simulink model "ModeAdjust"  (R2018b)
settings: Solver=FixedStepDiscrete  StartTime=0.0  StopTime=inf  FixedStep=0.01  RelTol=1e-3
undefined symbols (not defined in the file or in its folder): IfKeSMSbSeatMovBkRclnEnable_Val, IfKeSMSbSeatMovFrwdBkwdEnable_Val, IfKeSMSbSeatMovFtrstEnable_Val, IfKeSMSbSeatMovHdrstFrwdBkwdEnable_Val, IfKeSMSbSeatMovHdUpwdDnwdEnable_Val, IfKeSMSbSeatMovLgrstEnable_Val, IfKeSMSbSeatMovLtwdRtwdEnable_Val, IfVeSMSeStNumConfig, KeSMSbArmscreenMovEnable_Val, KeSMSbSeatMovLgrstExpdEnable_Val, KeSMSuFirstRwStBackPosDelta_Val, KeSMSuFirstRwStBackPosTolr_Val, KeSMSuFirstRwStCushFrntPosDelta_Val, KeSMSuFirstRwStCushFrntPosTolr_Val, KeSMSuFirstRwStCushRePosDelta_Val, KeSMSuFirstRwStCushRePosTolr_Val, KeSMSuFirstRwStFootrestPosDelta_Val, KeSMSuFirstRwStFootrestPosTolr_Val, KeSMSuFirstRwStFwdBkwdPosDelta_Val, KeSMSuFirstRwStFwdBkwdPosTolr_Val, KeSMSuMdMotFinshdTm_Val, KeSMSuMdRetryTm1_Val, KeSMSuModeReqDurgTm_Val, KeSMSuSecRwStArmTochPosDelta_Val, KeSMSuSecRwStArmTochPosTolr_Val, KeSMSuSecRwStBackPosDelta_Val, KeSMSuSecRwStBackPosTolr_Val, KeSMSuSecRwStFtrstUpwdDnwdPosDelta_Val, KeSMSuSecRwStFtrstUpwdDnwdPosTolr_Val, KeSMSuSecRwStFwdBkwdPosDelta_Val, KeSMSuSecRwStFwdBkwdPosTolr_Val, KeSMSuSecRwStHeadrestFwdBkwdPosDelta_Val, KeSMSuSecRwStHeadrestFwdBkwdPosTolr_Val, KeSMSuSecRwStHeadrestUpwdDwnwdPosDelta_Val, KeSMSuSecRwStHeadrestUpwdDwnwdPosTolr_Val, KeSMSuSecRwStLegrestInOutPosDelta_Val, KeSMSuSecRwStLegrestInOutPosTolr_Val, KeSMSuSecRwStLegrestUpwdDwnwdPosDelta_Val, KeSMSuSecRwStLegrestUpwdDwnwdPosTolr_Val, KeSMSuSecRwStLwdRwdPosDelta_Val, KeSMSuSecRwStLwdRwdPosTolr_Val, KeSMSuSecRwStVIPFtrstRefAngle_Val, KeSMSuThirdRwStFwdBkwdPosDelta_Val, KeSMSuThirdRwStFwdBkwdPosTolr_Val, KeSMSuThrdRwCushFoldPosDelta_Val, KeSMSuThrdRwCushFoldPosTolr_Val, KeSMSuThrdRwStBackPosDelta_Val, KeSMSuThrdRwStBackPosTolr_Val, KeSMSw4SLegrstCloseMdSecRwLtStFtrstUpwdDnwdPos_Val, KeSMSw4SLegrstCloseMdSecRwLtStFtrstUpwdDnwdPosMax_Val, KeSMSw4SLegrstCloseMdSecRwLtStFtrstUpwdDnwdPosMin_Val, KeSMSw4SLegrstCloseMdSecRwLtStLgrstOtwdInwdPos_Val, KeSMSw4SLegrstCloseMdSecRwLtStLgrstOtwdInwdPosMax_Val, KeSMSw4SLegrstCloseMdSecRwLtStLgrstOtwdInwdPosMin_Val, KeSMSw4SLegrstCloseMdSecRwLtStLgrstUpwdDnwdPos_Val, KeSMSw4SLegrstCloseMdSecRwLtStLgrstUpwdDnwdPosMax_Val, KeSMSw4SLegrstCloseMdSecRwLtStLgrstUpwdDnwdPosMin_Val, KeSMSw4SLegrstCloseMdSecRwRtStFtrstUpwdDnwdPos_Val, KeSMSw4SLegrstCloseMdSecRwRtStFtrstUpwdDnwdPosMax_Val, KeSMSw4SLegrstCloseMdSecRwRtStFtrstUpwdDnwdPosMin_Val ... (+1138)
libraries: Lib x401
(part 12 of 35)

== system ModeAdjust/ModeAdjustRunnable_sys/ModeAdjust/AcsMdEntry/R2Rt ==
  note: /*短期措施：二右扶手屏配置信号原先的短期措施blost inout被头枕前后占用，暂时默认扶手屏始终配置，等46数据库再连线*/
  note: %1锁，2未锁
  Mode_Trig : Inport
  Step1En : Inport  Port=2
  Step2En : Inport  Port=3
  SecRwRtStPoss : Inport  Port=4
  SecRwRtStPossV : Inport  Port=5
  SecRwRtStChldLkRsp_L : Inport  Port=6
  ModeStCalib_2R : Inport  Port=7
  StConfig : Inport  Port=8
  isR2RtSeatOccupied : Inport  Port=9
  AND : Logic  AllPortsSameDT=off  OutDataTypeStr=boolean
  Bus Creator : BusCreator  Inputs=9  OutDataTypeStr=Bus: SecRwRtSeatPos
  Bus Selector : BusSelector  OutputSignals=IfVeSMSuSecRwRtStBkReclnUpwdDnwdPos_Val_read,IfVeSMSuSecRwRtStFrwdBkwdPos_Val_read,IfVeSMSuSecRwRtStHPassStUpwdDnwdPos_Val_read,IfVeSMSuSecRwRtStLgrstUpwdDnwdPos_Val_read,IfVeSMSuSecRwRtStLtwdRtwdPos_Val_read,SecRwRtStArmScrnPos_Val_read
  Bus Selector1 : BusSelector  OutputSignals=IfVeSMSuSecRwRtStBkReclnUpwdDnwdPosV_Val_read,IfVeSMSuSecRwRtStFrwdBkwdPosV_Val_read,IfVeSMSuSecRwRtStHPassStUpwdDnwdPosV_Val_read,IfVeSMSuSecRwRtStLgrstUpwdDnwdPosV_Val_read,IfVeSMSuSecRwRtStLtwdRtwdPosV_Val_read,SecRwRtStArmScrnPosV_Val_read
  Bus Selector2 : BusSelector  OutputSignals=ArmScrnPos,ArmScrnPosMax,ArmScrnPosMin,BkReclnUpwdDnwdPos,BkReclnUpwdDnwdPosMax,BkReclnUpwdDnwdPosMin,FrwdBkwdPos,FrwdBkwdPosMax,FrwdBkwdPosMin,HdrstUpwdPos,HdrstUpwdPosMax,HdrstUpwdPosMin,LgrstUpwdPos,LgrstUpwdPosMax,LgrstUpwdPosMin,LtwdRtwdPos,LtwdRtwdPosMax,LtwdRtwdPosMin
  Bus Selector3 : BusSelector  OutputSignals=AcsEntrySecRwRtSt
  Bus Selector4 : BusSelector  OutputSignals=BkReclnUpwdDnwdMovConfig,ArmTouchMovConfig,FrwdBkwdMovConfig,LgrstUpwdMovConfig,LtwdRtwdMovConfig
  Logical Operator1 : Logic  Inputs=3  AllPortsSameDT=off  OutDataTypeStr=boolean
  Logical Operator2 : Logic  Inputs=3  AllPortsSameDT=off  OutDataTypeStr=boolean
  Logical Operator3 : Logic  AllPortsSameDT=off  OutDataTypeStr=boolean
  Logical Operator4 : Logic  AllPortsSameDT=off  OutDataTypeStr=boolean
  Logical Operator5 : Logic  Operator=OR  AllPortsSameDT=off  OutDataTypeStr=boolean
  Logical Operator6 : Logic  AllPortsSameDT=off  OutDataTypeStr=boolean
  NOT : Logic  Operator=NOT  AllPortsSameDT=off  OutDataTypeStr=boolean
  PA_KeSMSuMdMotFinshdTm_Val : Constant  Value=KeSMSuMdMotFinshdTm_Val
  PA_KeSMSuMdRetryTm1_Val : Constant  Value=KeSMSuMdRetryTm1_Val
  PA_KeSMSuModeReqDurgTm_Val : Constant  Value=KeSMSuModeReqDurgTm_Val
  PA_KeSMSuSecRwStArmTochPosDelta_Val : Constant  Value=KeSMSuSecRwStArmTochPosDelta_Val
  PA_KeSMSuSecRwStBackPosDelta_Val : Constant  Value=KeSMSuSecRwStBackPosDelta_Val
  PA_KeSMSuSecRwStFwdBkwdPosDelta_Val : Constant  Value=KeSMSuSecRwStFwdBkwdPosDelta_Val
  PA_KeSMSuSecRwStLegrestUpwdDwnwdPosDelta_Val : Constant  Value=KeSMSuSecRwStLegrestUpwdDwnwdPosDelta_Val
  PA_KeSMSuSecRwStLwdRwdPosDelta_Val : Constant  Value=KeSMSuSecRwStLwdRwdPosDelta_Val
  PA_KeSMSwDltTrgtPos_Val{1,4..5,7..9,11,14,16} (9 alike) : Constant  Value=0  OutDataTypeStr=boolean
  PA_KeSMSwDltTrgtPos_Val{3,6,10,12,15,17,19..22} (10 alike) : Constant  Value=KeSMSwPosInvalidVal_Val
  PA_KeSMSwDltTrgtPos_Val18 : Constant  Value=3  OutDataTypeStr=uint8
  PA_KeSMSwDltTrgtPos_Val2 : Constant  Value=SeatChldLkSt.ChldLkSt_Unlock
  PA_KeSMSwDltTrgtPos_Val23 : Constant  Value=2  OutDataTypeStr=uint8
  PA_KeSMSwSecRwRtStEasyEntryCllsnPt_Val : Constant  Value=KeSMSwSecRwRtStEasyEntryCllsnPt_Val
  R2RtSt_BkReclnUpwdDnwd_Step1 : Lib/CommonUsed  SystemSampleTime=-1
  R2RtSt_FrwdBkwd_Step2 : Lib/CommonUsed  SystemSampleTime=-1
  R2RtSt_LgrstUpwd_Step1 : Lib/CommonUsed  SystemSampleTime=-1
  R2Rt_LtwdRtwd_Step2 : Lib/CommonUsed  SystemSampleTime=-1
  Relational Operator : RelationalOperator  Operator=~=  OutDataTypeStr=boolean  RndMeth=Simplest
  Relational Operator1 : RelationalOperator  Operator=<=  OutDataTypeStr=boolean  RndMeth=Simplest
  Relational Operator2 : RelationalOperator  Operator=~=  OutDataTypeStr=boolean  RndMeth=Simplest
  SecRwRtStArmScrnPos_Step1 : Lib/CommonUsed  SystemSampleTime=-1
  Switch : Switch  Criteria=u2 ~= 0
  R2RtSt_Step1_ini : Outport
  R2RtSt_Step2_ini : Outport  Port=2
  R2Rt_Step1_done : Outport  Port=3
  R2Rt_Step2_done : Outport  Port=4
  R2Rt_TrgtPoss : Outport  Port=5  VectorParamsAs1DForOutWhenUnconnected=on
  R2Rt_SpdCtrl : Outport  Port=6
  wires:
  R2RtSt_LgrstUpwd_Step1/4 -> [Step1done_2]
  R2RtSt_LgrstUpwd_Step1/3 -> [R2RtSt_LgrstUpwd_TarPos]
  R2RtSt_LgrstUpwd_Step1/2 -> [Step1_2_ArrivedTarPos]
  [Tick] -> R2RtSt_LgrstUpwd_Step1/11
  PA_KeSMSwDltTrgtPos_Val12/1 -> R2RtSt_LgrstUpwd_Step1/10
  PA_KeSMSwDltTrgtPos_Val11/1 -> R2RtSt_LgrstUpwd_Step1/9
  [SecRwRtStLgrstUpwdDnwdPosV] -> R2RtSt_LgrstUpwd_Step1/8
  [KeSMSuSecRwStLegrestUpwdDwnwdPosDelta_Val] -> R2RtSt_LgrstUpwd_Step1/7
  [SecRwRtStBkReclnUpwdDnwdPosV] -> R2RtSt_BkReclnUpwdDnwd_Step1/8
  [SecRwRtStLgrstUpwdDnwdPos] -> R2RtSt_LgrstUpwd_Step1/3
  [K_LgrstUpwdPos] -> R2RtSt_LgrstUpwd_Step1/6
  [K_LgrstUpwdPosMax] -> R2RtSt_LgrstUpwd_Step1/5
  [K_LgrstUpwdPosMin] -> R2RtSt_LgrstUpwd_Step1/4
  [Step1En] -> R2RtSt_LgrstUpwd_Step1/2
  [Trig] -> R2RtSt_LgrstUpwd_Step1/1
  Relational Operator/1 -> [ChildLocker]
  PA_KeSMSwDltTrgtPos_Val2/1 -> Relational Operator/2
  SecRwRtStChldLkRsp_L/1 -> Relational Operator/1
  R2RtSt_FrwdBkwd_Step2/4 -> [Step2done_1]
  [Tick] -> R2RtSt_FrwdBkwd_Step2/11
  [Tick] -> R2RtSt_BkReclnUpwdDnwd_Step1/11
  PA_KeSMSwDltTrgtPos_Val6/1 -> R2RtSt_FrwdBkwd_Step2/10
  PA_KeSMSwDltTrgtPos_Val14/1 -> R2RtSt_FrwdBkwd_Step2/9
  [ChildLocker] -> R2RtSt_BkReclnUpwdDnwd_Step1/9
  [SecRwRtStFrwdBkwdPosV] -> R2RtSt_FrwdBkwd_Step2/8
  [K_FrwdBkwdPos] -> R2RtSt_FrwdBkwd_Step2/6
  [Step2En] -> R2RtSt_FrwdBkwd_Step2/2
  [Trig] -> R2RtSt_FrwdBkwd_Step2/1
  [Step1En] -> R2RtSt_BkReclnUpwdDnwd_Step1/2
  R2RtSt_BkReclnUpwdDnwd_Step1/4 -> [Step1done_1]
  R2RtSt_BkReclnUpwdDnwd_Step1/3 -> [R2RtSt_BkReclnUpwdDnwd_TarPos]
  PA_KeSMSwDltTrgtPos_Val3/1 -> R2RtSt_BkReclnUpwdDnwd_Step1/10
  [K_BkReclnUpwdDnwdPos] -> R2RtSt_BkReclnUpwdDnwd_Step1/6
  [SecRwRtStBkReclnUpwdDnwdPos] -> R2RtSt_BkReclnUpwdDnwd_Step1/3
  R2RtSt_BkReclnUpwdDnwd_Step1/2 -> [Step1_1_ArrivedTarPos]
  [K_BkReclnUpwdDnwdPosMin] -> R2RtSt_BkReclnUpwdDnwd_Step1/4
  R2RtSt_FrwdBkwd_Step2/2 -> [Step2_1_ArrivedTarPos]
  R2RtSt_FrwdBkwd_Step2/1 -> [FrwdBkwd_inidone_Step2]
  [K_FrwdBkwdPosMin] -> R2RtSt_FrwdBkwd_Step2/4
  [KeSMSuSecRwStFwdBkwdPosDelta_Val] -> R2RtSt_FrwdBkwd_Step2/7
  [K_FrwdBkwdPosMax] -> R2RtSt_FrwdBkwd_Step2/5
  [SecRwRtStFrwdBkwdPos] -> R2RtSt_FrwdBkwd_Step2/3
  [KeSMSuSecRwStBackPosDelta_Val] -> R2RtSt_BkReclnUpwdDnwd_Step1/7
  Mode_Trig/1 -> [Trig]
  [Trig] -> R2RtSt_BkReclnUpwdDnwd_Step1/1
  [K_BkReclnUpwdDnwdPosMax] -> R2RtSt_BkReclnUpwdDnwd_Step1/5
  Bus Selector1/2 -> [SecRwRtStFrwdBkwdPosV]  "<IfVeSMSuSecRwRtStFrwdBkwdPosV_Val_read>"
  SecRwRtStPossV/1 -> Bus Selector1/1
  Bus Selector1/3 -> [SecRwRtStHPassStUpwdDnwdPosV]  "<IfVeSMSuSecRwRtStHPassStUpwdDnwdPosV_Val_read>"
  Bus Selector/4 -> [SecRwRtStLgrstUpwdDnwdPos]  "<IfVeSMSuSecRwRtStLgrstUpwdDnwdPos_Val_read>"
  Bus Selector1/1 -> [SecRwRtStBkReclnUpwdDnwdPosV]  "<IfVeSMSuSecRwRtStBkReclnUpwdDnwdPosV_Val_read>"
  Bus Selector/1 -> [SecRwRtStBkReclnUpwdDnwdPos]  "<IfVeSMSuSecRwRtStBkReclnUpwdDnwdPos_Val_read>"
  Bus Selector1/4 -> [SecRwRtStLgrstUpwdDnwdPosV]  "<IfVeSMSuSecRwRtStLgrstUpwdDnwdPosV_Val_read>"
  Bus Selector/5 -> [SecRwRtStLtwdRtwdPos]  "<IfVeSMSuSecRwRtStLtwdRtwdPos_Val_read>"
  SecRwRtStPoss/1 -> Bus Selector/1
  Bus Selector1/5 -> [SecRwRtStLtwdRtwdPosV]  "<IfVeSMSuSecRwRtStLtwdRtwdPosV_Val_read>"
  Bus Selector/3 -> [SecRwRtStHPassStUpwdDnwdPos]  "<IfVeSMSuSecRwRtStHPassStUpwdDnwdPos_Val_read>"
  Bus Selector/2 -> [SecRwRtStFrwdBkwdPos]  "<IfVeSMSuSecRwRtStFrwdBkwdPos_Val_read>"
  [SecRwRtStArmScrnPos] -> SecRwRtStArmScrnPos_Step1/3
  [SecRwRtStArmScrnPosV] -> SecRwRtStArmScrnPos_Step1/8
  [Trig] -> SecRwRtStArmScrnPos_Step1/1
  [Step1En] -> SecRwRtStArmScrnPos_Step1/2
  [K_ArmScrnPosMin] -> SecRwRtStArmScrnPos_Step1/4
  [K_ArmScrnPosMax] -> SecRwRtStArmScrnPos_Step1/5
  [K_ArmScrnPos] -> SecRwRtStArmScrnPos_Step1/6
  PA_KeSMSwDltTrgtPos_Val7/1 -> SecRwRtStArmScrnPos_Step1/9
  PA_KeSMSwDltTrgtPos_Val10/1 -> SecRwRtStArmScrnPos_Step1/10
  [Tick] -> SecRwRtStArmScrnPos_Step1/11
  R2RtSt_FrwdBkwd_Step2/3 -> [R2Rt_StFrwdBkwd_TarPos]
  [Step1done_1] -> Logical Operator2/1
  [Step1done_2] -> Logical Operator2/2
  [Step1done_3] -> Logical Operator2/3
  [SecRwRtStFrwdBkwdPos] -> Relational Operator1/1
  [Trig] -> R2Rt_LtwdRtwd_Step2/1
  [Step2done_1] -> Logical Operator5/1
  Logical Operator5/1 -> Logical Operator4/1
  Logical Operator4/1 -> R2Rt_LtwdRtwd_Step2/2
  Relational Operator1/1 -> Logical Operator5/2
  [Step2En] -> Logical Operator4/2
  [KeSMSuSecRwStArmTochPosDelta_Val] -> SecRwRtStArmScrnPos_Step1/7
  [SecRwRtStLtwdRtwdPos] -> R2Rt_LtwdRtwd_Step2/3
  [SecRwRtStLtwdRtwdPosV] -> R2Rt_LtwdRtwd_Step2/8
  [K_LtwdRtwdPosMin] -> R2Rt_LtwdRtwd_Step2/4
  [K_LtwdRtwdPosMax] -> R2Rt_LtwdRtwd_Step2/5
  [K_LtwdRtwdPos] -> R2Rt_LtwdRtwd_Step2/6
  [KeSMSuSecRwStLwdRwdPosDelta_Val] -> R2Rt_LtwdRtwd_Step2/7
  PA_KeSMSwDltTrgtPos_Val16/1 -> R2Rt_LtwdRtwd_Step2/9
  PA_KeSMSwDltTrgtPos_Val17/1 -> R2Rt_LtwdRtwd_Step2/10
  [Tick] -> R2Rt_LtwdRtwd_Step2/11
  R2Rt_LtwdRtwd_Step2/3 -> [R2Rt_LtwdRtwd_TarPos]
  R2Rt_LtwdRtwd_Step2/1 -> [LtwdRtwd_inidone_Step2]
  R2Rt_LtwdRtwd_Step2/2 -> [Step2_2_ArrivedTarPos]
  R2Rt_LtwdRtwd_Step2/4 -> [Step2done_2]
  R2RtSt_BkReclnUpwdDnwd_Step1/1 -> [ReclnUpwdDnwd_Step1_ini]
  R2RtSt_LgrstUpwd_Step1/1 -> [LgrstUpwd_Step1_ini]
  [ReclnUpwdDnwd_Step1_ini] -> Logical Operator1/1
  [LgrstUpwd_Step1_ini] -> Logical Operator1/2
  [LtStArmScrn_Step1_ini] -> Logical Operator1/3
  Logical Operator1/1 -> R2RtSt_Step1_ini/1
  [FrwdBkwd_inidone_Step2] -> Logical Operator6/1
  [LtwdRtwd_inidone_Step2] -> Logical Operator6/2
  Logical Operator6/1 -> R2RtSt_Step2_ini/1
  Logical Operator2/1 -> R2Rt_Step1_done/1
  [Step2done_1] -> Logical Operator3/1
  [Step2done_2] -> Logical Operator3/2
  Logical Operator3/1 -> R2Rt_Step2_done/1
  Bus Creator/1 -> R2Rt_TrgtPoss/1
  [R2Rt_StFrwdBkwd_TarPos] -> Bus Creator/5  "SecRwRtStFrwdBkwdTrgtPos"
  [R2Rt_LtwdRtwd_TarPos] -> Bus Creator/8  "SecRwRtStLtwdRtwdTrgtPos"
  PA_KeSMSwDltTrgtPos_Val22/1 -> Bus Creator/6  "SecRwRtStHdrstUpwdDnwdTrgtPos"
  [R2RtSt_LgrstUpwd_TarPos] -> Bus Creator/7  "SecRwRtStLgrstUpwdDnwdTrgtPos"
  PA_KeSMSwDltTrgtPos_Val19/1 -> Bus Creator/2  "SecRwRtStBlstOtwdInwdTrgtPos"
  [R2RtSt_BkReclnUpwdDnwd_TarPos] -> Bus Creator/1  "SecRwRtStBkReclnUpwdDnwdTrgtPos"
  PA_KeSMSwDltTrgtPos_Val20/1 -> Bus Creator/3  "SecRwRtStCshnFrntUpwdDnwdTrgtPos"
  PA_KeSMSwDltTrgtPos_Val21/1 -> Bus Creator/4  "SecRwRtStCshnRrUpwdDnwdTrgtPos"
  Step1En/1 -> [Step1En]
  Step2En/1 -> [Step2En]
  PA_KeSMSuModeReqDurgTm_Val/1 -> [Tick]
  [SecRwRtStArmScrnTrgtPos] -> Bus Creator/9  "SecRwRtStArmScrnTrgtPos"
  SecRwRtStArmScrnPos_Step1/1 -> [LtStArmScrn_Step1_ini]
  SecRwRtStArmScrnPos_Step1/2 -> [Step1_3_ArrivedTarPos]
  SecRwRtStArmScrnPos_Step1/3 -> [SecRwRtStArmScrnTrgtPos]
  SecRwRtStArmScrnPos_Step1/4 -> [Step1done_3]
  PA_KeSMSuSecRwStFwdBkwdPosDelta_Val/1 -> [KeSMSuSecRwStFwdBkwdPosDelta_Val]
  PA_KeSMSuSecRwStLwdRwdPosDelta_Val/1 -> [KeSMSuSecRwStLwdRwdPosDelta_Val]
  PA_KeSMSuSecRwStLegrestUpwdDwnwdPosDelta_Val/1 -> [KeSMSuSecRwStLegrestUpwdDwnwdPosDelta_Val]
  PA_KeSMSuMdMotFinshdTm_Val/1 -> [KeSMSuMdMotFinshdTm_Val]
  PA_KeSMSuSecRwStBackPosDelta_Val/1 -> [KeSMSuSecRwStBackPosDelta_Val]
  PA_KeSMSuSecRwStArmTochPosDelta_Val/1 -> [KeSMSuSecRwStArmTochPosDelta_Val]
  [KeSMSuMdMotFinshdTm_Val] -> R2RtSt_BkReclnUpwdDnwd_Step1/12
  [KeSMSuMdMotFinshdTm_Val] -> R2RtSt_LgrstUpwd_Step1/12
  [KeSMSuMdMotFinshdTm_Val] -> SecRwRtStArmScrnPos_Step1/12
  [KeSMSuMdMotFinshdTm_Val] -> R2RtSt_FrwdBkwd_Step2/12
  [KeSMSuMdMotFinshdTm_Val] -> R2Rt_LtwdRtwd_Step2/12
  Bus Selector/6 -> [SecRwRtStArmScrnPos]  "<SecRwRtStArmScrnPos_Val_read>"
  Bus Selector1/6 -> [SecRwRtStArmScrnPosV]  "<SecRwRtStArmScrnPosV_Val_read>"
  PA_KeSMSwSecRwRtStEasyEntryCllsnPt_Val/1 -> Relational Operator1/2
  Bus Selector2/1 -> [K_ArmScrnPos]  "<ArmScrnPos>"
  Bus Selector2/18 -> [K_LtwdRtwdPosMin]  "<LtwdRtwdPosMin>"
  Bus Selector2/16 -> [K_LtwdRtwdPos]  "<LtwdRtwdPos>"
  Bus Selector2/15 -> [K_LgrstUpwdPosMin]  "<LgrstUpwdPosMin>"
  Bus Selector2/17 -> [K_LtwdRtwdPosMax]  "<LtwdRtwdPosMax>"
  Bus Selector2/12 -> [K_HdrstUpwdPosMin]  "<HdrstUpwdPosMin>"
  Bus Selector2/13 -> [K_LgrstUpwdPos]  "<LgrstUpwdPos>"
  Bus Selector2/11 -> [K_HdrstUpwdPosMax]  "<HdrstUpwdPosMax>"
  Bus Selector2/14 -> [K_LgrstUpwdPosMax]  "<LgrstUpwdPosMax>"
  Bus Selector2/10 -> [K_HdrstUpwdPos]  "<HdrstUpwdPos>"
  Bus Selector2/4 -> [K_BkReclnUpwdDnwdPos]  "<BkReclnUpwdDnwdPos>"
  Bus Selector2/9 -> [K_FrwdBkwdPosMin]  "<FrwdBkwdPosMin>"
  Bus Selector2/5 -> [K_BkReclnUpwdDnwdPosMax]  "<BkReclnUpwdDnwdPosMax>"
  Bus Selector2/8 -> [K_FrwdBkwdPosMax]  "<FrwdBkwdPosMax>"
  Bus Selector3/1 -> Bus Selector2/1  "<AcsEntrySecRwRtSt>"
  Bus Selector2/7 -> [K_FrwdBkwdPos]  "<FrwdBkwdPos>"
  Bus Selector2/3 -> [K_ArmScrnPosMin]  "<ArmScrnPosMin>"
  Bus Selector2/2 -> [K_ArmScrnPosMax]  "<ArmScrnPosMax>"
  Bus Selector2/6 -> [K_BkReclnUpwdDnwdPosMin]  "<BkReclnUpwdDnwdPosMin>"
  ModeStCalib_2R/1 -> Bus Selector3/1
  PA_KeSMSwDltTrgtPos_Val1/1 -> R2RtSt_LgrstUpwd_Step1/13
  PA_KeSMSwDltTrgtPos_Val4/1 -> R2RtSt_FrwdBkwd_Step2/13
  PA_KeSMSwDltTrgtPos_Val5/1 -> R2Rt_LtwdRtwd_Step2/13
  PA_KeSMSwDltTrgtPos_Val8/1 -> SecRwRtStArmScrnPos_Step1/13
  PA_KeSMSwDltTrgtPos_Val9/1 -> R2RtSt_BkReclnUpwdDnwd_Step1/13
  StConfig/1 -> Bus Selector4/1
  Bus Selector4/1 -> [BkReclnUpwdDnwdMovConfig]  "<BkReclnUpwdDnwdMovConfig>"
  Bus Selector4/2 -> [ArmTouchMovConfig]  "<ArmTouchMovConfig>"
  Bus Selector4/3 -> [FrwdBkwdMovConfig]  "<FrwdBkwdMovConfig>"
  Bus Selector4/4 -> [LgrstUpwdMovConfig]  "<LgrstUpwdMovConfig>"
  Bus Selector4/5 -> [LtwdRtwdMovConfig]  "<LtwdRtwdMovConfig>"
  [LgrstUpwdMovConfig] -> R2RtSt_LgrstUpwd_Step1/14
  [BkReclnUpwdDnwdMovConfig] -> R2RtSt_BkReclnUpwdDnwd_Step1/14
  [LtwdRtwdMovConfig] -> R2Rt_LtwdRtwd_Step2/14
  [FrwdBkwdMovConfig] -> R2RtSt_FrwdBkwd_Step2/14
  [ArmTouchMovConfig] -> SecRwRtStArmScrnPos_Step1/14
  [CntLow] -> R2RtSt_BkReclnUpwdDnwd_Step1/15
  [CntLow] -> R2RtSt_FrwdBkwd_Step2/15
  [CntLow] -> R2RtSt_LgrstUpwd_Step1/15
  [CntLow] -> R2Rt_LtwdRtwd_Step2/15
  [CntLow] -> SecRwRtStArmScrnPos_Step1/15
  PA_KeSMSuMdRetryTm1_Val/1 -> [CntLow]
  isR2RtSeatOccupied/1 -> NOT/1
  NOT/1 -> AND/1
  PA_KeSMSwDltTrgtPos_Val23/1 -> Switch/3
  PA_KeSMSwDltTrgtPos_Val15/1 -> Relational Operator2/2  "SecRwLtStHdrstUpwdDnwdTrgtPos"
  [R2Rt_StFrwdBkwd_TarPos] -> Relational Operator2/1  "SecRwLtStFrwdBkwdTrgtPos"
  PA_KeSMSwDltTrgtPos_Val18/1 -> Switch/1
  AND/1 -> Switch/2
  Switch/1 -> R2Rt_SpdCtrl/1
  Relational Operator2/1 -> AND/2

== system ModeAdjust/ModeAdjustRunnable_sys/ModeAdjust/AcsMdEntry/R3Lt ==
  Mode_Trig : Inport
  Step1En : Inport  Port=2
  Step2En : Inport  Port=3
  Step3En : Inport  Port=4
  isSeatOccupied : Inport  Port=5
  ThdRwLtStPoss : Inport  Port=6
  ThdRwLtStPossV : Inport  Port=7
  ModeStCalib_3L : Inport  Port=8
  is6s : Inport  Port=9
  StConfig : Inport  Port=10
  isR2LtSeatOccupied : Inport  Port=11
  isR2RtSeatOccupied : Inport  Port=12
  AND : Logic  AllPortsSameDT=off  OutDataTypeStr=boolean
  AND1 : Logic  Operator=OR  AllPortsSameDT=off  OutDataTypeStr=boolean
  AND2 : Logic  AllPortsSameDT=off  OutDataTypeStr=boolean
  Bus Creator : BusCreator  Inputs=3  OutDataTypeStr=Bus: ThdRwLfSeatPos
  Bus Selector : BusSelector  OutputSignals=IfVeSMSuThdRwLtStBkReclnUpwdDnwdPos_Val_read,IfVeSMSuThdRwLtStCshnFldUpwdDnwdPos_Val_read,IfVeSMSuThdRwLtStFrwdBkwdPos_Val_read
  Bus Selector1 : BusSelector  OutputSignals=IfVeSMSuThdRwLtStBkReclnUpwdDnwdPosV_Val_read,IfVeSMSuThdRwLtStCshnFldUpwdDnwdPosV_Val_read,IfVeSMSuThdRwLtStFrwdBkwdPosV_Val_read
  Bus Selector2 : BusSelector  OutputSignals=BkReclnUpwdDnwdPos,BkReclnUpwdDnwdPosMax,BkReclnUpwdDnwdPosMin,CshnFldUpwdDnwdPos,CshnFldUpwdDnwdPosMax,CshnFldUpwdDnwdPosMin,FrwdBkwdPos,FrwdBkwdPosMax,FrwdBkwdPosMin
  Bus Selector3 : BusSelector  OutputSignals=AcsEntryThdRwLtSt
  Bus Selector4 : BusSelector  OutputSignals=BkReclnUpwdDnwdMovConfig,CshnFldUpwdDnwdMovConfig,FrwdBkwdMovConfig
  NOT : Logic  Operator=NOT  AllPortsSameDT=off  OutDataTypeStr=boolean
  NOT1 : Logic  Operator=NOT  AllPortsSameDT=off  OutDataTypeStr=boolean
  NOT2 : Logic  Operator=NOT  AllPortsSameDT=off  OutDataTypeStr=boolean
  PA_KeSMSuMdMotFinshdTm_Val : Constant  Value=KeSMSuMdMotFinshdTm_Val
  PA_KeSMSuMdRetryTm1_Val : Constant  Value=KeSMSuMdRetryTm1_Val
  PA_KeSMSuModeReqDurgTm_Val : Constant  Value=KeSMSuModeReqDurgTm_Val
  PA_KeSMSuThirdRwStFwdBkwdPosDelta_Val : Constant  Value=KeSMSuThirdRwStFwdBkwdPosDelta_Val
  PA_KeSMSuThrdRwCushFoldPosDelta_Val : Constant  Value=KeSMSuThrdRwCushFoldPosDelta_Val
  PA_KeSMSuThrdRwStBackPosDelta_Val : Constant  Value=KeSMSuThrdRwStBackPosDelta_Val
  PA_KeSMSwDltTrgtPos_Val10 : Constant  OutDataTypeStr=boolean
  PA_KeSMSwDltTrgtPos_Val{3,6..7,15} (4 alike) : Constant  Value=KeSMSwPosInvalidVal_Val
  PA_KeSMSwDltTrgtPos_Val2 : Constant  Value=0  OutDataTypeStr=boolean
  PA_KeSMSwDltTrgtPos_Val22 : Constant  Value=3  OutDataTypeStr=uint8
  PA_KeSMSwDltTrgtPos_Val23 : Constant  Value=2  OutDataTypeStr=uint8
  PA_KeSMSwDltTrgtPos_Val4 : Constant  Value=0  OutDataTypeStr=boolean
  PA_KeSMSwDltTrgtPos_Val9 : Constant  Value=0  OutDataTypeStr=boolean
  R3LtSt_BkReclnUpwdDnwd_Step1 : Lib/CommonUsed  SystemSampleTime=-1
  R3Lt_CshnFldUpwdDnwd_Step3 : Lib/CommonUsed  SystemSampleTime=-1
  R3Lt_FrwdBkwd_Step2 : Lib/CommonUsed  SystemSampleTime=-1
  Relational Operator2 : RelationalOperator  Operator=~=  OutDataTypeStr=boolean  RndMeth=Simplest
  Switch : Switch  Criteria=u2 > Threshold
  Switch1 : Switch  Criteria=u2 ~= 0
  R3Lt_Step1_ini : Outport
  R3Lt_Step2_ini : Outport  Port=2
  R3Lt_Step3_ini : Outport  Port=3
  EZE_R3Lt_BkReclnUpwdDnwd_Movedone_Step1 : Outport  Port=4
  EZE_R3LtFrwdBkwd_Movedone_Step2 : Outport  Port=5
  EZE_R3Lt_CshnFldUpwdDnwd_MovedoneStep3 : Outport  Port=6
  IfVeSMSbThdRwLtStRclCmdSrv_Val_writeRaw : Outport  Port=7
  R3Lt_TrgtPoss : Outport  Port=8  VectorParamsAs1DForOutWhenUnconnected=on
  R3Lt_SpdCtrl : Outport  Port=9
  wires:
  R3Lt_CshnFldUpwdDnwd_Step3/4 -> [Step3done], EZE_R3Lt_CshnFldUpwdDnwd_MovedoneStep3/1
  R3Lt_CshnFldUpwdDnwd_Step3/3 -> [R3Lt_CshnFldUpwdDnwd_TarPos]
  [ThdRwLtStCshnFldUpwdDnwdPosV] -> R3Lt_CshnFldUpwdDnwd_Step3/8
  [Tick] -> R3Lt_CshnFldUpwdDnwd_Step3/11
  PA_KeSMSwDltTrgtPos_Val7/1 -> R3Lt_CshnFldUpwdDnwd_Step3/10
  [isSeatOccupied] -> R3Lt_CshnFldUpwdDnwd_Step3/9
  Step3En/1 -> R3Lt_CshnFldUpwdDnwd_Step3/2
  [Trig] -> R3Lt_CshnFldUpwdDnwd_Step3/1
  R3Lt_FrwdBkwd_Step2/4 -> [Step2done], EZE_R3LtFrwdBkwd_Movedone_Step2/1
  R3Lt_FrwdBkwd_Step2/3 -> [R3LtFrwdBkwd_TarPos]
  [Tick] -> R3Lt_FrwdBkwd_Step2/11
  [Tick] -> R3LtSt_BkReclnUpwdDnwd_Step1/11
  PA_KeSMSwDltTrgtPos_Val6/1 -> R3Lt_FrwdBkwd_Step2/10
  [isSeatOccupied] -> R3Lt_FrwdBkwd_Step2/9
  [isSeatOccupied] -> R3LtSt_BkReclnUpwdDnwd_Step1/9
  isSeatOccupied/1 -> [isSeatOccupied]
  [ThdRwLtStFrwdBkwdPosV] -> R3Lt_FrwdBkwd_Step2/8
  [K_FrwdBkwdPos] -> R3Lt_FrwdBkwd_Step2/6
  Step2En/1 -> R3Lt_FrwdBkwd_Step2/2
  [Trig] -> R3Lt_FrwdBkwd_Step2/1
  Step1En/1 -> R3LtSt_BkReclnUpwdDnwd_Step1/2
  R3LtSt_BkReclnUpwdDnwd_Step1/4 -> [Step1done], EZE_R3Lt_BkReclnUpwdDnwd_Movedone_Step1/1
  R3LtSt_BkReclnUpwdDnwd_Step1/3 -> [R3Lt_BkReclnUpwdDnwd_TarPos]
  PA_KeSMSwDltTrgtPos_Val3/1 -> R3LtSt_BkReclnUpwdDnwd_Step1/10
  [ThdRwLtStBkReclnUpwdDnwdPosV] -> R3LtSt_BkReclnUpwdDnwd_Step1/8
  [K_BkReclnUpwdDnwdPos] -> R3LtSt_BkReclnUpwdDnwd_Step1/6
  [K_CshnFldUpwdDnwdPosMin] -> R3Lt_CshnFldUpwdDnwd_Step3/4
  [ThdRwLtStBkReclnUpwdDnwdPos] -> R3LtSt_BkReclnUpwdDnwd_Step1/3
  R3LtSt_BkReclnUpwdDnwd_Step1/2 -> [Step1ArrivedTarPos]
  [K_BkReclnUpwdDnwdPosMin] -> R3LtSt_BkReclnUpwdDnwd_Step1/4
  R3Lt_FrwdBkwd_Step2/2 -> [Step2ArrivedTarPos]
  R3Lt_FrwdBkwd_Step2/1 -> R3Lt_Step2_ini/1
  [KeSMSuThrdRwCushFoldPosDelta_Val] -> R3Lt_CshnFldUpwdDnwd_Step3/7
  R3LtSt_BkReclnUpwdDnwd_Step1/1 -> R3Lt_Step1_ini/1
  [K_FrwdBkwdPosMin] -> R3Lt_FrwdBkwd_Step2/4
  [KeSMSuThirdRwStFwdBkwdPosDelta_Val] -> R3Lt_FrwdBkwd_Step2/7
  [K_CshnFldUpwdDnwdPos] -> R3Lt_CshnFldUpwdDnwd_Step3/6
  R3Lt_CshnFldUpwdDnwd_Step3/1 -> R3Lt_Step3_ini/1
  [K_FrwdBkwdPosMax] -> R3Lt_FrwdBkwd_Step2/5
  [ThdRwLtStCshnFldUpwdDnwdPos] -> R3Lt_CshnFldUpwdDnwd_Step3/3
  [ThdRwLtStFrwdBkwdPos] -> R3Lt_FrwdBkwd_Step2/3
  [KeSMSuThrdRwStBackPosDelta_Val] -> R3LtSt_BkReclnUpwdDnwd_Step1/7
  [K_CshnFldUpwdDnwdPosMax] -> R3Lt_CshnFldUpwdDnwd_Step3/5
  Mode_Trig/1 -> [Trig]
  R3Lt_CshnFldUpwdDnwd_Step3/2 -> [Step3ArrivedTarPos]
  [Trig] -> R3LtSt_BkReclnUpwdDnwd_Step1/1
  [K_BkReclnUpwdDnwdPosMax] -> R3LtSt_BkReclnUpwdDnwd_Step1/5
  [isSeatOccupied] -> Switch/2
  Switch/1 -> IfVeSMSbThdRwLtStRclCmdSrv_Val_writeRaw/1
  PA_KeSMSwDltTrgtPos_Val9/1 -> Switch/1
  PA_KeSMSwDltTrgtPos_Val10/1 -> Switch/3
  Bus Selector/2 -> [ThdRwLtStCshnFldUpwdDnwdPos]  "<IfVeSMSuThdRwLtStCshnFldUpwdDnwdPos_Val_read>"
  Bus Selector1/2 -> [ThdRwLtStCshnFldUpwdDnwdPosV]  "<IfVeSMSuThdRwLtStCshnFldUpwdDnwdPosV_Val_read>"
  ThdRwLtStPoss/1 -> Bus Selector/1
  Bus Selector/3 -> [ThdRwLtStFrwdBkwdPos]  "<IfVeSMSuThdRwLtStFrwdBkwdPos_Val_read>"
  Bus Selector1/3 -> [ThdRwLtStFrwdBkwdPosV]  "<IfVeSMSuThdRwLtStFrwdBkwdPosV_Val_read>"
  ThdRwLtStPossV/1 -> Bus Selector1/1
  Bus Selector1/1 -> [ThdRwLtStBkReclnUpwdDnwdPosV]  "<IfVeSMSuThdRwLtStBkReclnUpwdDnwdPosV_Val_read>"
  Bus Selector/1 -> [ThdRwLtStBkReclnUpwdDnwdPos]  "<IfVeSMSuThdRwLtStBkReclnUpwdDnwdPos_Val_read>"
  [R3LtFrwdBkwd_TarPos] -> Bus Creator/3  "ThdRwLtStFrwdBkwdTrgtPos"
  [R3Lt_CshnFldUpwdDnwd_TarPos] -> Bus Creator/2  "ThdRwLtStCshnFldUpwdDnwdTrgtPos"
  [R3Lt_BkReclnUpwdDnwd_TarPos] -> Bus Creator/1  "ThdRwLtStBkReclnUpwdDnwdTrgtPos"
  Bus Creator/1 -> R3Lt_TrgtPoss/1
  PA_KeSMSuMdMotFinshdTm_Val/1 -> [KeSMSuMdMotFinshdTm_Val]
  PA_KeSMSuThrdRwStBackPosDelta_Val/1 -> [KeSMSuThrdRwStBackPosDelta_Val]
  PA_KeSMSuThirdRwStFwdBkwdPosDelta_Val/1 -> [KeSMSuThirdRwStFwdBkwdPosDelta_Val]
  PA_KeSMSuThrdRwCushFoldPosDelta_Val/1 -> [KeSMSuThrdRwCushFoldPosDelta_Val]
  PA_KeSMSuModeReqDurgTm_Val/1 -> [Tick]
  [KeSMSuMdMotFinshdTm_Val] -> R3LtSt_BkReclnUpwdDnwd_Step1/12
  [KeSMSuMdMotFinshdTm_Val] -> R3Lt_FrwdBkwd_Step2/12
  [KeSMSuMdMotFinshdTm_Val] -> R3Lt_CshnFldUpwdDnwd_Step3/12
  Bus Selector2/1 -> [K_BkReclnUpwdDnwdPos]  "<BkReclnUpwdDnwdPos>"
  Bus Selector2/9 -> [K_FrwdBkwdPosMin]  "<FrwdBkwdPosMin>"
  Bus Selector2/2 -> [K_BkReclnUpwdDnwdPosMax]  "<BkReclnUpwdDnwdPosMax>"
  Bus Selector2/8 -> [K_FrwdBkwdPosMax]  "<FrwdBkwdPosMax>"
  Bus Selector3/1 -> Bus Selector2/1  "<AcsEntryThdRwLtSt>"
  Bus Selector2/7 -> [K_FrwdBkwdPos]  "<FrwdBkwdPos>"
  Bus Selector2/3 -> [K_BkReclnUpwdDnwdPosMin]  "<BkReclnUpwdDnwdPosMin>"
  ModeStCalib_3L/1 -> Bus Selector3/1
  Bus Selector2/4 -> [K_CshnFldUpwdDnwdPos]  "<CshnFldUpwdDnwdPos>"
  Bus Selector2/5 -> [K_CshnFldUpwdDnwdPosMax]  "<CshnFldUpwdDnwdPosMax>"
  Bus Selector2/6 -> [K_CshnFldUpwdDnwdPosMin]  "<CshnFldUpwdDnwdPosMin>"
  is6s/1 -> [is6s]
  [is6s] -> R3Lt_CshnFldUpwdDnwd_Step3/13
  PA_KeSMSwDltTrgtPos_Val2/1 -> R3LtSt_BkReclnUpwdDnwd_Step1/13
  PA_KeSMSwDltTrgtPos_Val4/1 -> R3Lt_FrwdBkwd_Step2/13
  StConfig/1 -> Bus Selector4/1
  Bus Selector4/1 -> [BkReclnUpwdDnwdMovConfig]  "<BkReclnUpwdDnwdMovConfig>"
  Bus Selector4/2 -> [CshnFldUpwdDnwdMovConfig]  "<CshnFldUpwdDnwdMovConfig>"
  Bus Selector4/3 -> [FrwdBkwdMovConfig]  "<FrwdBkwdMovConfig>"
  [FrwdBkwdMovConfig] -> R3Lt_FrwdBkwd_Step2/14
  [CshnFldUpwdDnwdMovConfig] -> R3Lt_CshnFldUpwdDnwd_Step3/14
  [BkReclnUpwdDnwdMovConfig] -> R3LtSt_BkReclnUpwdDnwd_Step1/14
  [CntLow] -> R3LtSt_BkReclnUpwdDnwd_Step1/15
  [CntLow] -> R3Lt_CshnFldUpwdDnwd_Step3/15
  [CntLow] -> R3Lt_FrwdBkwd_Step2/15
  PA_KeSMSuMdRetryTm1_Val/1 -> [CntLow]
  isR2LtSeatOccupied/1 -> NOT/1
  PA_KeSMSwDltTrgtPos_Val23/1 -> Switch1/3
  PA_KeSMSwDltTrgtPos_Val15/1 -> Relational Operator2/2  "SecRwLtStHdrstUpwdDnwdTrgtPos"
  [R3LtFrwdBkwd_TarPos] -> Relational Operator2/1  "SecRwLtStFrwdBkwdTrgtPos"
  PA_KeSMSwDltTrgtPos_Val22/1 -> Switch1/1
  AND/1 -> Switch1/2
  Switch1/1 -> R3Lt_SpdCtrl/1
  Relational Operator2/1 -> AND/2
  isR2RtSeatOccupied/1 -> NOT1/1
  NOT1/1 -> AND2/2
  NOT2/1 -> AND2/1
  AND1/1 -> AND/1
  NOT/1 -> AND1/2
  AND2/1 -> AND1/1
  [is6s] -> NOT2/1

== system ModeAdjust/ModeAdjustRunnable_sys/ModeAdjust/AcsMdEntry/R3Rt ==
  Mode_Trig : Inport
  Step1En : Inport  Port=2
  Step2En : Inport  Port=3
  Step3En : Inport  Port=4
  SeatOccupied : Inport  Port=5
  ThdRwRtStPoss : Inport  Port=6
  ThdRwRtStPossV : Inport  Port=7
  ModeStCalib_3R : Inport  Port=8
  is6s : Inport  Port=9
  StConfig : Inport  Port=10
  isR2RtSeatOccupied : Inport  Port=11
  AND : Logic  AllPortsSameDT=off  OutDataTypeStr=boolean
  Bus Creator : BusCreator  Inputs=3  OutDataTypeStr=Bus: ThdRwRtSeatPos
  Bus Selector : BusSelector  OutputSignals=IfVeSMSuThdRwRtStBkReclnUpwdDnwdPos_Val_read,IfVeSMSuThdRwRtStCshnFldUpwdDnwdPos_Val_read,IfVeSMSuThdRwRtStFrwdBkwdPos_Val_read
  Bus Selector1 : BusSelector  OutputSignals=IfVeSMSuThdRwRtStBkReclnUpwdDnwdPosV_Val_read,IfVeSMSuThdRwRtStCshnFldUpwdDnwdPosV_Val_read,IfVeSMSuThdRwRtStFrwdBkwdPosV_Val_read
  Bus Selector2 : BusSelector  OutputSignals=BkReclnUpwdDnwdPos,BkReclnUpwdDnwdPosMax,BkReclnUpwdDnwdPosMin,CshnFldUpwdDnwdPos,CshnFldUpwdDnwdPosMax,CshnFldUpwdDnwdPosMin,FrwdBkwdPos,FrwdBkwdPosMax,FrwdBkwdPosMin
  Bus Selector3 : BusSelector  OutputSignals=AcsEntryThdRwRtSt
  Bus Selector4 : BusSelector  OutputSignals=BkReclnUpwdDnwdMovConfig,CshnFldUpwdDnwdMovConfig,FrwdBkwdMovConfig
  NOT : Logic  Operator=NOT  AllPortsSameDT=off  OutDataTypeStr=boolean
  PA_KeSMSuMdMotFinshdTm_Val : Constant  Value=KeSMSuMdMotFinshdTm_Val
  PA_KeSMSuMdRetryTm1_Val : Constant  Value=KeSMSuMdRetryTm1_Val
  PA_KeSMSuModeReqDurgTm_Val : Constant  Value=KeSMSuModeReqDurgTm_Val
  PA_KeSMSuThirdRwStFwdBkwdPosDelta_Val : Constant  Value=KeSMSuThirdRwStFwdBkwdPosDelta_Val
  PA_KeSMSuThrdRwCushFoldPosDelta_Val : Constant  Value=KeSMSuThrdRwCushFoldPosDelta_Val
  PA_KeSMSuThrdRwStBackPosDelta_Val : Constant  Value=KeSMSuThrdRwStBackPosDelta_Val
  PA_KeSMSwDltTrgtPos_Val10 : Constant  OutDataTypeStr=boolean
  PA_KeSMSwDltTrgtPos_Val{3,6..7,15} (4 alike) : Constant  Value=KeSMSwPosInvalidVal_Val
  PA_KeSMSwDltTrgtPos_Val2 : Constant  Value=0  OutDataTypeStr=boolean
  PA_KeSMSwDltTrgtPos_Val22 : Constant  Value=3  OutDataTypeStr=uint8
  PA_KeSMSwDltTrgtPos_Val23 : Constant  Value=2  OutDataTypeStr=uint8
  PA_KeSMSwDltTrgtPos_Val4 : Constant  Value=0  OutDataTypeStr=boolean
  PA_KeSMSwDltTrgtPos_Val9 : Constant  Value=0  OutDataTypeStr=boolean
  R3RtReclnUpDn_Step1 : Lib/CommonUsed  SystemSampleTime=-1
  R3Rt_CshnFldUpwdDnwd_Step3 : Lib/CommonUsed  SystemSampleTime=-1
  R3Rt_FrwdBkwd_Step2 : Lib/CommonUsed  SystemSampleTime=-1
  Relational Operator2 : RelationalOperator  Operator=~=  OutDataTypeStr=boolean  RndMeth=Simplest
  Switch : Switch  Criteria=u2 > Threshold
  Switch1 : Switch  Criteria=u2 ~= 0
  R3Rt_Step1_ini : Outport
  R3Rt_Step2_ini : Outport  Port=2
  R3Rt_Step3_ini : Outport  Port=3
  EZE_R3RtReclnUpDn_Movedone_Step1 : Outport  Port=4
  EZE_R3Rt_FrwdBkwd_Movedone_Step2 : Outport  Port=5
  EZE_R3Rt_CshnFldUpwdDnwd_Movedone_Step3 : Outport  Port=6
  IfVeSMSbThdRwRtStRclCmdSrv_Val_writeRaw : Outport  Port=7
  R3Rt_TrgtPoss : Outport  Port=8  VectorParamsAs1DForOutWhenUnconnected=on
  R3Rt_SpdCtrl : Outport  Port=9
  wires:
  [K_BkReclnUpwdDnwdPosMax] -> R3RtReclnUpDn_Step1/5
  [Trig] -> R3RtReclnUpDn_Step1/1
  R3Rt_CshnFldUpwdDnwd_Step3/2 -> [Step3ArrivedTarPos]
  Mode_Trig/1 -> [Trig]
  [K_CshnFldUpwdDnwdPosMax] -> R3Rt_CshnFldUpwdDnwd_Step3/5
  [KeSMSuThrdRwStBackPosDelta_Val] -> R3RtReclnUpDn_Step1/7
  [ThdRwRtStFrwdBkwdPos] -> R3Rt_FrwdBkwd_Step2/3
  [ThdRwRtStCshnFldUpwdDnwdPos] -> R3Rt_CshnFldUpwdDnwd_Step3/3
  [K_FrwdBkwdPosMax] -> R3Rt_FrwdBkwd_Step2/5
  R3Rt_CshnFldUpwdDnwd_Step3/1 -> R3Rt_Step3_ini/1
  [K_CshnFldUpwdDnwdPos] -> R3Rt_CshnFldUpwdDnwd_Step3/6
  [KeSMSuThirdRwStFwdBkwdPosDelta_Val] -> R3Rt_FrwdBkwd_Step2/7
  [K_FrwdBkwdPosMin] -> R3Rt_FrwdBkwd_Step2/4
  [KeSMSuThrdRwCushFoldPosDelta_Val] -> R3Rt_CshnFldUpwdDnwd_Step3/7
  R3Rt_FrwdBkwd_Step2/1 -> R3Rt_Step2_ini/1
  R3Rt_FrwdBkwd_Step2/2 -> [Step2ArrivedTarPos]
  [K_BkReclnUpwdDnwdPosMin] -> R3RtReclnUpDn_Step1/4
  R3RtReclnUpDn_Step1/2 -> [Step1ArrivedTarPos]
  [ThdRwRtStBkReclnUpwdDnwdPos] -> R3RtReclnUpDn_Step1/3
  [K_CshnFldUpwdDnwdPosMin] -> R3Rt_CshnFldUpwdDnwd_Step3/4
  [K_BkReclnUpwdDnwdPos] -> R3RtReclnUpDn_Step1/6
  [ThdRwRtStBkReclnUpwdDnwdPosV] -> R3RtReclnUpDn_Step1/8
  PA_KeSMSwDltTrgtPos_Val3/1 -> R3RtReclnUpDn_Step1/10
  R3RtReclnUpDn_Step1/3 -> [R3RtReclnUpDn_TarPos]
  R3RtReclnUpDn_Step1/4 -> EZE_R3RtReclnUpDn_Movedone_Step1/1
  Step1En/1 -> R3RtReclnUpDn_Step1/2
  [Trig] -> R3Rt_FrwdBkwd_Step2/1
  Step2En/1 -> R3Rt_FrwdBkwd_Step2/2
  [K_FrwdBkwdPos] -> R3Rt_FrwdBkwd_Step2/6
  [ThdRwRtStFrwdBkwdPosV] -> R3Rt_FrwdBkwd_Step2/8
  SeatOccupied/1 -> [isSeatOccupied]
  [isSeatOccupied] -> R3RtReclnUpDn_Step1/9
  [isSeatOccupied] -> R3Rt_FrwdBkwd_Step2/9
  PA_KeSMSwDltTrgtPos_Val6/1 -> R3Rt_FrwdBkwd_Step2/10
  [Tick] -> R3RtReclnUpDn_Step1/11
  [Tick] -> R3Rt_FrwdBkwd_Step2/11
  R3Rt_FrwdBkwd_Step2/3 -> [R3Rt_FrwdBkwd_TarPos]
  R3Rt_FrwdBkwd_Step2/4 -> EZE_R3Rt_FrwdBkwd_Movedone_Step2/1, [Step2done]
  [Trig] -> R3Rt_CshnFldUpwdDnwd_Step3/1
  Step3En/1 -> R3Rt_CshnFldUpwdDnwd_Step3/2
  [isSeatOccupied] -> R3Rt_CshnFldUpwdDnwd_Step3/9
  PA_KeSMSwDltTrgtPos_Val7/1 -> R3Rt_CshnFldUpwdDnwd_Step3/10
  [Tick] -> R3Rt_CshnFldUpwdDnwd_Step3/11
  [ThdRwRtStCshnFldUpwdDnwdPosV] -> R3Rt_CshnFldUpwdDnwd_Step3/8
  R3Rt_CshnFldUpwdDnwd_Step3/3 -> [R3Rt_CshnFldUpwdDnwd_TarPos]
  R3Rt_CshnFldUpwdDnwd_Step3/4 -> [Step3done], EZE_R3Rt_CshnFldUpwdDnwd_Movedone_Step3/1
  [isSeatOccupied] -> Switch/2
  PA_KeSMSwDltTrgtPos_Val9/1 -> Switch/1
  PA_KeSMSwDltTrgtPos_Val10/1 -> Switch/3
  Switch/1 -> IfVeSMSbThdRwRtStRclCmdSrv_Val_writeRaw/1
  Bus Selector1/1 -> [ThdRwRtStBkReclnUpwdDnwdPosV]  "<IfVeSMSuThdRwRtStBkReclnUpwdDnwdPosV_Val_read>"
  Bus Selector/3 -> [ThdRwRtStFrwdBkwdPos]  "<IfVeSMSuThdRwRtStFrwdBkwdPos_Val_read>"
  ThdRwRtStPossV/1 -> Bus Selector1/1
  ThdRwRtStPoss/1 -> Bus Selector/1
  Bus Selector/2 -> [ThdRwRtStCshnFldUpwdDnwdPos]  "<IfVeSMSuThdRwRtStCshnFldUpwdDnwdPos_Val_read>"
  Bus Selector/1 -> [ThdRwRtStBkReclnUpwdDnwdPos]  "<IfVeSMSuThdRwRtStBkReclnUpwdDnwdPos_Val_read>"
  Bus Selector1/2 -> [ThdRwRtStCshnFldUpwdDnwdPosV]  "<IfVeSMSuThdRwRtStCshnFldUpwdDnwdPosV_Val_read>"
  Bus Selector1/3 -> [ThdRwRtStFrwdBkwdPosV]  "<IfVeSMSuThdRwRtStFrwdBkwdPosV_Val_read>"
  R3RtReclnUpDn_Step1/1 -> R3Rt_Step1_ini/1
  [R3Rt_CshnFldUpwdDnwd_TarPos] -> Bus Creator/2  "ThdRwRtStCshnFldUpwdDnwdTrgtPos"
  [R3RtReclnUpDn_TarPos] -> Bus Creator/1  "ThdRwRtStBkReclnUpwdDnwdTrgtPos"
  [R3Rt_FrwdBkwd_TarPos] -> Bus Creator/3  "ThdRwRtStFrwdBkwdTrgtPos"
  Bus Creator/1 -> R3Rt_TrgtPoss/1
  PA_KeSMSuModeReqDurgTm_Val/1 -> [Tick]
  PA_KeSMSuMdMotFinshdTm_Val/1 -> [KeSMSuMdMotFinshdTm_Val]
  PA_KeSMSuThrdRwStBackPosDelta_Val/1 -> [KeSMSuThrdRwStBackPosDelta_Val]
  PA_KeSMSuThirdRwStFwdBkwdPosDelta_Val/1 -> [KeSMSuThirdRwStFwdBkwdPosDelta_Val]
  PA_KeSMSuThrdRwCushFoldPosDelta_Val/1 -> [KeSMSuThrdRwCushFoldPosDelta_Val]
  [KeSMSuMdMotFinshdTm_Val] -> R3RtReclnUpDn_Step1/12
  [KeSMSuMdMotFinshdTm_Val] -> R3Rt_FrwdBkwd_Step2/12
  [KeSMSuMdMotFinshdTm_Val] -> R3Rt_CshnFldUpwdDnwd_Step3/12
  Bus Selector2/6 -> [K_CshnFldUpwdDnwdPosMin]  "<CshnFldUpwdDnwdPosMin>"
  Bus Selector2/4 -> [K_CshnFldUpwdDnwdPos]  "<CshnFldUpwdDnwdPos>"
  Bus Selector2/7 -> [K_FrwdBkwdPos]  "<FrwdBkwdPos>"
  Bus Selector2/5 -> [K_CshnFldUpwdDnwdPosMax]  "<CshnFldUpwdDnwdPosMax>"
  ModeStCalib_3R/1 -> Bus Selector3/1
  Bus Selector2/3 -> [K_BkReclnUpwdDnwdPosMin]  "<BkReclnUpwdDnwdPosMin>"
  Bus Selector3/1 -> Bus Selector2/1  "<AcsEntryThdRwRtSt>"
  Bus Selector2/9 -> [K_FrwdBkwdPosMin]  "<FrwdBkwdPosMin>"
  Bus Selector2/2 -> [K_BkReclnUpwdDnwdPosMax]  "<BkReclnUpwdDnwdPosMax>"
  Bus Selector2/1 -> [K_BkReclnUpwdDnwdPos]  "<BkReclnUpwdDnwdPos>"
  Bus Selector2/8 -> [K_FrwdBkwdPosMax]  "<FrwdBkwdPosMax>"
  is6s/1 -> [is6s]
  [is6s] -> R3Rt_CshnFldUpwdDnwd_Step3/13
  PA_KeSMSwDltTrgtPos_Val2/1 -> R3Rt_FrwdBkwd_Step2/13
  PA_KeSMSwDltTrgtPos_Val4/1 -> R3RtReclnUpDn_Step1/13
  Bus Selector4/1 -> [BkReclnUpwdDnwdMovConfig]  "<BkReclnUpwdDnwdMovConfig>"
  StConfig/1 -> Bus Selector4/1
  Bus Selector4/2 -> [CshnFldUpwdDnwdMovConfig]  "<CshnFldUpwdDnwdMovConfig>"
  Bus Selector4/3 -> [FrwdBkwdMovConfig]  "<FrwdBkwdMovConfig>"
  [CshnFldUpwdDnwdMovConfig] -> R3Rt_CshnFldUpwdDnwd_Step3/14
  [FrwdBkwdMovConfig] -> R3Rt_FrwdBkwd_Step2/14
  [BkReclnUpwdDnwdMovConfig] -> R3RtReclnUpDn_Step1/14
  [CntLow] -> R3RtReclnUpDn_Step1/15
  [CntLow] -> R3Rt_CshnFldUpwdDnwd_Step3/15
  [CntLow] -> R3Rt_FrwdBkwd_Step2/15
  PA_KeSMSuMdRetryTm1_Val/1 -> [CntLow]
  isR2RtSeatOccupied/1 -> NOT/1
  NOT/1 -> AND/1
  PA_KeSMSwDltTrgtPos_Val23/1 -> Switch1/3
  PA_KeSMSwDltTrgtPos_Val15/1 -> Relational Operator2/2  "SecRwLtStHdrstUpwdDnwdTrgtPos"
  [R3Rt_FrwdBkwd_TarPos] -> Relational Operator2/1  "SecRwLtStFrwdBkwdTrgtPos"
  PA_KeSMSwDltTrgtPos_Val22/1 -> Switch1/1
  AND/1 -> Switch1/2
  Switch1/1 -> R3Rt_SpdCtrl/1
  Relational Operator2/1 -> AND/2

== system ModeAdjust/ModeAdjustRunnable_sys/ModeAdjust/AcsMdExt/Drv ==
  Mode_Trig : Inport
  Step1En : Inport  Port=2
  DrvCurPos : Inport  Port=3
  DrvCurPosV : Inport  Port=4
  ModeStCalib_Drv : Inport  Port=5
  StConfig : Inport  Port=6
  Bus Creator : BusCreator  Inputs=8  OutDataTypeStr=Bus: DrvSeatPos
  Bus Selector : BusSelector  OutputSignals=IfVeSMSuDrvStFtUpwdDnwdPos_Val_read,IfVeSMSuDrvStBkReclnUpwdDnwdPos_Val_read,IfVeSMSuDrvStCshnFrntUpwdDnwdPos_Val_read,IfVeSMSuDrvStCshnRrUpwdDnwdPos_Val_read,IfVeSMSuDrvStFrwdBkwdPos_Val_read
  Bus Selector1 : BusSelector  OutputSignals=IfVeSMSuDrvStFtUpwdDnwdPosV_Val_read,IfVeSMSuDrvStBkReclnUpwdDnwdPosV_Val_read,IfVeSMSuDrvStCshnFrntUpwdDnwdPosV_Val_read,IfVeSMSuDrvStCshnRrUpwdDnwdPosV_Val_read,IfVeSMSuDrvStFrwdBkwdPosV_Val_read
  Bus Selector2 : BusSelector  OutputSignals=BkReclnUpwdDnwdPos,BkReclnUpwdDnwdPosMax,BkReclnUpwdDnwdPosMin,FrwdBkwdPos,FrwdBkwdPosMax,FrwdBkwdPosMin,FtUpwdDnwdPos,FtUpwdDnwdPosMax,FtUpwdDnwdPosMin
  Bus Selector3 : BusSelector  OutputSignals=AcsExtDrvSt
  Bus Selector4 : BusSelector  OutputSignals=BkReclnUpwdDnwdMovConfig,FrwdBkwdMovConfig,FtUpwdDnwdMovConfig
  FtUpwdDnwd : Lib/CommonUsed  SystemSampleTime=-1
  PA_KeSMSuFirstRwStBackPosDelta_Val : Constant  Value=KeSMSuFirstRwStBackPosDelta_Val
  PA_KeSMSuFirstRwStFootrestPosDelta_Val : Constant  Value=KeSMSuFirstRwStFootrestPosDelta_Val
  PA_KeSMSuFirstRwStFwdBkwdPosDelta_Val : Constant  Value=KeSMSuFirstRwStFwdBkwdPosDelta_Val
  PA_KeSMSuMdMotFinshdTm_Val : Constant  Value=KeSMSuMdMotFinshdTm_Val
  PA_KeSMSuMdRetryTm1_Val : Constant  Value=KeSMSuMdRetryTm1_Val
  PA_KeSMSuModeReqDurgTm_Val : Constant  Value=KeSMSuModeReqDurgTm_Val
  PA_KeSMSwDltTrgtPos_Val1 : Constant  Value=0  OutDataTypeStr=boolean
  PA_KeSMSwDltTrgtPos_Val{2..3,10,12..16} (8 alike) : Constant  Value=KeSMSwPosInvalidVal_Val
  PA_KeSMSwDltTrgtPos_Val11 : Constant  Value=0  OutDataTypeStr=boolean
  PA_KeSMSwDltTrgtPos_Val17 : Constant  OutDataTypeStr=boolean
  DrvSt_Step1_ini : Outport
  DrvSt_Step1_done : Outport  Port=2
  EZE_DrvStTrgtPoss : Outport  Port=3  VectorParamsAs1DForOutWhenUnconnected=on
  IfVeSMSbDrvStRclCmdSrv_Val_writeRaw : Outport  Port=4
  wires:
  PA_KeSMSwDltTrgtPos_Val2/1 -> Bus Creator/8  "DrvStFrwdBkwdTrgtPos"
  PA_KeSMSwDltTrgtPos_Val15/1 -> Bus Creator/6  "DrvStCshnFrntUpwdDnwdTrgtPos"
  Bus Creator/1 -> EZE_DrvStTrgtPoss/1
  [DrvSt_FtUpwdDnwd_TarPos] -> Bus Creator/2  "DrvStFtUpwdDnwdTrgtPos"
  PA_KeSMSwDltTrgtPos_Val13/1 -> Bus Creator/3  "DrvStHdrstUpwdDnwdTrgtPos"
  PA_KeSMSwDltTrgtPos_Val16/1 -> Bus Creator/7  "DrvStCshnRrUpwdDnwdTrgtPos"
  PA_KeSMSwDltTrgtPos_Val10/1 -> Bus Creator/1  "DrvStBlstOtwdInwdTrgtPos"
  PA_KeSMSwDltTrgtPos_Val3/1 -> Bus Creator/5  "DrvStBkReclnUpwdDnwdTrgtPos"
  PA_KeSMSwDltTrgtPos_Val14/1 -> Bus Creator/4  "DrvStLgrstUpwdDnwdTrgtPos"
  [FtUpwdDnwd_Step1_ini] -> DrvSt_Step1_ini/1
  [Step1done_2] -> DrvSt_Step1_done/1, [Step1done]
  Bus Selector/5 -> [DrvStFrwdBkwdPos]  "<IfVeSMSuDrvStFrwdBkwdPos_Val_read>"
  Bus Selector/3 -> [DrvStCshnFrntUpwdDnwdPos]  "<IfVeSMSuDrvStCshnFrntUpwdDnwdPos_Val_read>"
  DrvCurPos/1 -> Bus Selector/1
  Bus Selector1/5 -> [DrvStFrwdBkwdPosV]  "<IfVeSMSuDrvStFrwdBkwdPosV_Val_read>"
  DrvCurPosV/1 -> Bus Selector1/1
  Bus Selector1/3 -> [DrvStCshnFrntUpwdDnwdPosV]  "<IfVeSMSuDrvStCshnFrntUpwdDnwdPosV_Val_read>"
  Bus Selector1/4 -> [DrvStCshnRrUpwdDnwdPosV]  "<IfVeSMSuDrvStCshnRrUpwdDnwdPosV_Val_read>"
  Bus Selector/1 -> [DrvStFtUpwdDnwdPos]  "<IfVeSMSuDrvStFtUpwdDnwdPos_Val_read>"
  Bus Selector/2 -> [DrvStBkReclnUpwdDnwdPos]  "<IfVeSMSuDrvStBkReclnUpwdDnwdPos_Val_read>"
  Bus Selector1/2 -> [DrvStBkReclnUpwdDnwdPosV]  "<IfVeSMSuDrvStBkReclnUpwdDnwdPosV_Val_read>"
  Bus Selector/4 -> [DrvStCshnRrUpwdDnwdPos]  "<IfVeSMSuDrvStCshnRrUpwdDnwdPos_Val_read>"
  Bus Selector1/1 -> [DrvStFtUpwdDnwdPosV]  "<IfVeSMSuDrvStFtUpwdDnwdPosV_Val_read>"
  Mode_Trig/1 -> [Trig]
  [Trig] -> FtUpwdDnwd/1
  [Step1En] -> FtUpwdDnwd/2
  [K_DrvStFtUpwdDnwdPosMin] -> FtUpwdDnwd/4
  [K_DrvStFtUpwdDnwdPosMax] -> FtUpwdDnwd/5
  [K_DrvStFtUpwdDnwdPos] -> FtUpwdDnwd/6
  [DrvStFtUpwdDnwdPos] -> FtUpwdDnwd/3
  [KeSMSuFirstRwStFootrestPosDelta_Val] -> FtUpwdDnwd/7
  [DrvStFtUpwdDnwdPosV] -> FtUpwdDnwd/8
  PA_KeSMSwDltTrgtPos_Val11/1 -> FtUpwdDnwd/9
  PA_KeSMSwDltTrgtPos_Val12/1 -> FtUpwdDnwd/10
  [Tick] -> FtUpwdDnwd/11
  FtUpwdDnwd/1 -> [FtUpwdDnwd_Step1_ini]
  FtUpwdDnwd/2 -> [Step1_2_ArrivedTarPos]
  FtUpwdDnwd/3 -> [DrvSt_FtUpwdDnwd_TarPos]
  FtUpwdDnwd/4 -> [Step1done_2]
  Step1En/1 -> [Step1En]
  PA_KeSMSwDltTrgtPos_Val17/1 -> IfVeSMSbDrvStRclCmdSrv_Val_writeRaw/1
  PA_KeSMSuModeReqDurgTm_Val/1 -> [Tick]
  PA_KeSMSuFirstRwStBackPosDelta_Val/1 -> [KeSMSuFirstRwStBackPosDelta_Val]
  PA_KeSMSuFirstRwStFwdBkwdPosDelta_Val/1 -> [KeSMSuFirstRwStFwdBkwdPosDelta_Val]
  PA_KeSMSuMdMotFinshdTm_Val/1 -> [KeSMSuMdMotFinshdTm_Val]
  PA_KeSMSuFirstRwStFootrestPosDelta_Val/1 -> [KeSMSuFirstRwStFootrestPosDelta_Val]
  [KeSMSuMdMotFinshdTm_Val] -> FtUpwdDnwd/12
  Bus Selector2/4 -> [K_DrvStFrwdBkwdPos]  "<FrwdBkwdPos>"
  Bus Selector2/5 -> [K_DrvStFrwdBkwdPosMax]  "<FrwdBkwdPosMax>"
  Bus Selector2/7 -> [K_DrvStFtUpwdDnwdPos]  "<FtUpwdDnwdPos>"
  Bus Selector2/3 -> [K_DrvStBkReclnUpwdDnwdPosMin]  "<BkReclnUpwdDnwdPosMin>"
  Bus Selector2/8 -> [K_DrvStFtUpwdDnwdPosMax]  "<FtUpwdDnwdPosMax>"
  Bus Selector2/1 -> [K_DrvStBkReclnUpwdDnwdPos]  "<BkReclnUpwdDnwdPos>"
  Bus Selector2/9 -> [K_DrvStFtUpwdDnwdPosMin]  "<FtUpwdDnwdPosMin>"
  Bus Selector2/6 -> [K_DrvStFrwdBkwdPosMin]  "<FrwdBkwdPosMin>"
  Bus Selector3/1 -> Bus Selector2/1  "<AcsExtDrvSt>"
  ModeStCalib_Drv/1 -> Bus Selector3/1
  Bus Selector2/2 -> [K_DrvStBkReclnUpwdDnwdPosMax]  "<BkReclnUpwdDnwdPosMax>"
  PA_KeSMSwDltTrgtPos_Val1/1 -> FtUpwdDnwd/13
  Bus Selector4/1 -> [BkReclnUpwdDnwdMovConfig]  "<BkReclnUpwdDnwdMovConfig>"
  Bus Selector4/3 -> [FtUpwdDnwdMovConfig]  "<FtUpwdDnwdMovConfig>"
  Bus Selector4/2 -> [FrwdBkwdMovConfig]  "<FrwdBkwdMovConfig>"
  StConfig/1 -> Bus Selector4/1
  [FtUpwdDnwdMovConfig] -> FtUpwdDnwd/14
  [CntLow] -> FtUpwdDnwd/15
  PA_KeSMSuMdRetryTm1_Val/1 -> [CntLow]

== system ModeAdjust/ModeAdjustRunnable_sys/ModeAdjust/AcsMdExt/Pass ==
  Mode_Trig : Inport
  Step1En : Inport  Port=2
  PassStPoss : Inport  Port=3
  PassStPossV : Inport  Port=4
  ModeStCalib_Pass : Inport  Port=5
  StConfig : Inport  Port=6
  Bus Creator : BusCreator  Inputs=8  OutDataTypeStr=Bus: PasSeatPos
  Bus Selector : BusSelector  OutputSignals=IfVeSMSuPassStBkReclnUpwdDnwdPos_Val_read,IfVeSMSuPassStCshnFrntUpwdDnwdPos_Val_read,IfVeSMSuPassStCshnRrUpwdDnwdPos_Val_read,IfVeSMSuPassStFrwdBkwdPos_Val_read,IfVeSMSuPassStFtUpwdDnwdPos_Val_read
  Bus Selector1 : BusSelector  OutputSignals=IfVeSMSuPassStBkReclnUpwdDnwdPosV_Val_read,IfVeSMSuPassStCshnFrntUpwdDnwdPosV_Val_read,IfVeSMSuPassStCshnRrUpwdDnwdPosV_Val_read,IfVeSMSuPassStFrwdBkwdPosV_Val_read,IfVeSMSuPassStFtUpwdDnwdPosV_Val_read
  Bus Selector2 : BusSelector  OutputSignals=BkReclnUpwdDnwdPos,BkReclnUpwdDnwdPosMax,BkReclnUpwdDnwdPosMin,FrwdBkwdPos,FrwdBkwdPosMax,FrwdBkwdPosMin,FtUpwdDnwdPos,FtUpwdDnwdPosMax,FtUpwdDnwdPosMin
  Bus Selector3 : BusSelector  OutputSignals=AcsExtPassSt
  Bus Selector4 : BusSelector  OutputSignals=BkReclnUpwdDnwdMovConfig,FrwdBkwdMovConfig,FtUpwdDnwdMovConfig
  PA_KeSMSuFirstRwStBackPosDelta_Val : Constant  Value=KeSMSuFirstRwStBackPosDelta_Val
  PA_KeSMSuFirstRwStFootrestPosDelta_Val : Constant  Value=KeSMSuFirstRwStFootrestPosDelta_Val
  PA_KeSMSuFirstRwStFwdBkwdPosDelta_Val : Constant  Value=KeSMSuFirstRwStFwdBkwdPosDelta_Val
  PA_KeSMSuMdMotFinshdTm_Val : Constant  Value=KeSMSuMdMotFinshdTm_Val
  PA_KeSMSuMdRetryTm1_Val : Constant  Value=KeSMSuMdRetryTm1_Val
  PA_KeSMSuModeReqDurgTm_Val : Constant  Value=KeSMSuModeReqDurgTm_Val
  PA_KeSMSwDltTrgtPos_Val{1..2,12,14..18} (8 alike) : Constant  Value=KeSMSwPosInvalidVal_Val
  PA_KeSMSwDltTrgtPos_Val11 : Constant  Value=0  OutDataTypeStr=boolean
  PA_KeSMSwDltTrgtPos_Val4 : Constant  Value=0  OutDataTypeStr=boolean
  PA_KeSMSwDltTrgtPos_Val7 : Constant  OutDataTypeStr=boolean
  PassStFtUpwdDnwd_Step1 : Lib/CommonUsed  SystemSampleTime=-1
  Pass_Step1_ini : Outport
  Pass_Step1_done : Outport  Port=2
  PassStTrgtPoss : Outport  Port=3  VectorParamsAs1DForOutWhenUnconnected=on
  IfVeSMSuPassStRclCmdSrv_Val_writeRaw : Outport  Port=4
  wires:
  [PassStFtUpwdDnwd_TarPos] -> Bus Creator/6  "PassStFtUpwdDnwdTrgtPos"
  PA_KeSMSwDltTrgtPos_Val15/1 -> Bus Creator/3  "PassStCshnFrntUpwdDnwdTrgtPos"
  PA_KeSMSwDltTrgtPos_Val14/1 -> Bus Creator/2  "PassStBlstOtwdInwdTrgtPos"
  PA_KeSMSwDltTrgtPos_Val2/1 -> Bus Creator/1  "PassStBkReclnUpwdDnwdTrgtPos"
  PA_KeSMSwDltTrgtPos_Val18/1 -> Bus Creator/8  "PassStLgrstUpwdDnwdTrgtPos"
  PA_KeSMSwDltTrgtPos_Val17/1 -> Bus Creator/7  "PassStHdrstUpwdDnwdTrgtPos"
  PA_KeSMSwDltTrgtPos_Val1/1 -> Bus Creator/5  "PassStFrwdBkwdTrgtPos"
  PA_KeSMSwDltTrgtPos_Val16/1 -> Bus Creator/4  "PassStCshnRrUpwdDnwdTrgtPos"
  Bus Creator/1 -> PassStTrgtPoss/1
  [Step1done_2] -> Pass_Step1_done/1
  [FtUpwdDnwd_Step1_ini] -> Pass_Step1_ini/1
  PassStFtUpwdDnwd_Step1/1 -> [FtUpwdDnwd_Step1_ini]
  Bus Selector1/5 -> [PassStFtUpwdDnwdPosV]  "<IfVeSMSuPassStFtUpwdDnwdPosV_Val_read>"
  PassStPoss/1 -> Bus Selector/1
  Bus Selector1/1 -> [PassStBkReclnUpwdDnwdPosV]  "<IfVeSMSuPassStBkReclnUpwdDnwdPosV_Val_read>"
  Bus Selector1/4 -> [PassStFrwdBkwdPosV]  "<IfVeSMSuPassStFrwdBkwdPosV_Val_read>"
  Bus Selector/4 -> [PassStFrwdBkwdPos]  "<IfVeSMSuPassStFrwdBkwdPos_Val_read>"
  Bus Selector/1 -> [PassStBkReclnUpwdDnwdPos]  "<IfVeSMSuPassStBkReclnUpwdDnwdPos_Val_read>"
  Bus Selector1/2 -> [PassStCshnFrntUpwdDnwdPosV]  "<IfVeSMSuPassStCshnFrntUpwdDnwdPosV_Val_read>"
  Bus Selector/3 -> [PassStCshnRrUpwdDnwdPos]  "<IfVeSMSuPassStCshnRrUpwdDnwdPos_Val_read>"
  PassStPossV/1 -> Bus Selector1/1
  Bus Selector1/3 -> [PassStCshnRrUpwdDnwdPosV]  "<IfVeSMSuPassStCshnRrUpwdDnwdPosV_Val_read>"
  Bus Selector/5 -> [PassStFtUpwdDnwdPos]  "<IfVeSMSuPassStFtUpwdDnwdPos_Val_read>"
  Bus Selector/2 -> [PassStCshnFrntUpwdDnwdPos]  "<IfVeSMSuPassStCshnFrntUpwdDnwdPos_Val_read>"
  PassStFtUpwdDnwd_Step1/4 -> [Step1done_2]
  PassStFtUpwdDnwd_Step1/3 -> [PassStFtUpwdDnwd_TarPos]
  PassStFtUpwdDnwd_Step1/2 -> [Step1_2_ArrivedTarPos]
  [Tick] -> PassStFtUpwdDnwd_Step1/11
  PA_KeSMSwDltTrgtPos_Val12/1 -> PassStFtUpwdDnwd_Step1/10
  PA_KeSMSwDltTrgtPos_Val11/1 -> PassStFtUpwdDnwd_Step1/9
  [PassStFtUpwdDnwdPosV] -> PassStFtUpwdDnwd_Step1/8
  [KeSMSuFirstRwStFootrestPosDelta_Val] -> PassStFtUpwdDnwd_Step1/7
  [PassStFtUpwdDnwdPos] -> PassStFtUpwdDnwd_Step1/3
  [K_FtUpwdDnwdPos] -> PassStFtUpwdDnwd_Step1/6
  [K_FtUpwdDnwdPosMax] -> PassStFtUpwdDnwd_Step1/5
  [K_FtUpwdDnwdPosMin] -> PassStFtUpwdDnwd_Step1/4
  [Step1En] -> PassStFtUpwdDnwd_Step1/2
  [Trig] -> PassStFtUpwdDnwd_Step1/1
  Mode_Trig/1 -> [Trig]
  Step1En/1 -> [Step1En]
  PA_KeSMSwDltTrgtPos_Val7/1 -> IfVeSMSuPassStRclCmdSrv_Val_writeRaw/1
  PA_KeSMSuModeReqDurgTm_Val/1 -> [Tick]
  PA_KeSMSuFirstRwStBackPosDelta_Val/1 -> [KeSMSuFirstRwStBackPosDelta_Val]
  PA_KeSMSuFirstRwStFwdBkwdPosDelta_Val/1 -> [KeSMSuFirstRwStFwdBkwdPosDelta_Val]
  PA_KeSMSuMdMotFinshdTm_Val/1 -> [KeSMSuMdMotFinshdTm_Val]
  PA_KeSMSuFirstRwStFootrestPosDelta_Val/1 -> [KeSMSuFirstRwStFootrestPosDelta_Val]
  [KeSMSuMdMotFinshdTm_Val] -> PassStFtUpwdDnwd_Step1/12
  Bus Selector2/2 -> [K_BkReclnUpwdDnwdPosMax]  "<BkReclnUpwdDnwdPosMax>"
  Bus Selector2/9 -> [K_FtUpwdDnwdPosMin]  "<FtUpwdDnwdPosMin>"
  Bus Selector3/1 -> Bus Selector2/1  "<AcsExtPassSt>"
  ModeStCalib_Pass/1 -> Bus Selector3/1
  Bus Selector2/6 -> [K_FrwdBkwdPosMin]  "<FrwdBkwdPosMin>"
  Bus Selector2/3 -> [K_BkReclnUpwdDnwdPosMin]  "<BkReclnUpwdDnwdPosMin>"
  Bus Selector2/4 -> [K_FrwdBkwdPos]  "<FrwdBkwdPos>"
  Bus Selector2/7 -> [K_FtUpwdDnwdPos]  "<FtUpwdDnwdPos>"
  Bus Selector2/5 -> [K_FrwdBkwdPosMax]  "<FrwdBkwdPosMax>"
  Bus Selector2/1 -> [K_BkReclnUpwdDnwdPos]  "<BkReclnUpwdDnwdPos>"
  Bus Selector2/8 -> [K_FtUpwdDnwdPosMax]  "<FtUpwdDnwdPosMax>"
  PA_KeSMSwDltTrgtPos_Val4/1 -> PassStFtUpwdDnwd_Step1/13
  Bus Selector4/1 -> [BkReclnUpwdDnwdMovConfig]  "<BkReclnUpwdDnwdMovConfig>"
  Bus Selector4/3 -> [FtUpwdDnwdMovConfig]  "<FtUpwdDnwdMovConfig>"
  Bus Selector4/2 -> [FrwdBkwdMovConfig]  "<FrwdBkwdMovConfig>"
  StConfig/1 -> Bus Selector4/1
  [FtUpwdDnwdMovConfig] -> PassStFtUpwdDnwd_Step1/14
  [CntLow] -> PassStFtUpwdDnwd_Step1/15
  PA_KeSMSuMdRetryTm1_Val/1 -> [CntLow]
